simulink model "fullCarModel"  (R2024b)
settings: Solver=ode45  StartTime=0.0  StopTime=10.0  RelTol=1e-3  EnableMultiTasking=on
undefined symbols (not defined in the file or in its folder): sigbuilder_block
(part 2 of 2)

== system fullCarModel/vehicleBodyWith4Wheels/FullVehicle/wheelFR/FxfN/alfaFrontNew ==
  delta : Inport
  yVelo : Inport  Port=2
  Lf : Inport  Port=3
  yawRate : Inport  Port=4
  xVelo : Inport  Port=5
  Add : Sum  Inputs=+-
  Add1 : Sum
  Divide : Product  Inputs=*/
  Product : Product  RndMeth=Zero
  alfaFront : Outport
  wires:
  Lf/1 -> Product/1
  yawRate/1 -> Product/2
  Product/1 -> Add1/2
  yVelo/1 -> Add1/1
  Add1/1 -> Divide/1
  Divide/1 -> Add/2
  delta/1 -> Add/1
  Add/1 -> alfaFront/1
  xVelo/1 -> Divide/2

== system fullCarModel/vehicleBodyWith4Wheels/FullVehicle/wheelFR/FxfN/fLemda ==
  lamda : Inport
  Add : Sum  Inputs=+-
  Constant : Constant  Value=2
  Constant1 : Constant
  If : If  IfExpression=u1< 1  ZeroCross=off
  If Action Subsystem : Subsystem  TreatAsAtomicUnit=on
  If Action Subsystem1 : Subsystem  TreatAsAtomicUnit=on
  Merge : Merge
  Product : Product  RndMeth=Zero
  f_lamda : Outport
  wires:
  lamda/1 -> If/1, Add/2, Product/2
  If/1 -> If Action Subsystem1/Action
  If/2 -> If Action Subsystem/Action
  Constant/1 -> Add/1
  Add/1 -> Product/1
  Product/1 -> If Action Subsystem1/1(In1)
  Constant1/1 -> If Action Subsystem/1(In1)
  If Action Subsystem1/1(Out1) -> Merge/1
  If Action Subsystem/1(Out1) -> Merge/2
  Merge/1 -> f_lamda/1

== system fullCarModel/vehicleBodyWith4Wheels/FullVehicle/wheelFR/FxfN/lemda1 ==
  miu : Inport
  Fz : Inport  Port=2
  C_sigma : Inport  Port=3
  C_alfa : Inport  Port=4
  sigma : Inport  Port=5
  alfa : Inport  Port=6
  Add : Sum
  Add1 : Sum
  Constant : Constant  Value=2
  Constant1 : Constant
  Divide : Product  Inputs=*/
  Math Function : Math  Operator=square  SignedPower=on
  Math Function1 : Math  Operator=square  SignedPower=on
  Product{,1..4} (5 alike) : Product  RndMeth=Zero
  Sqrt : Sqrt
  Trigonometric Function : Trigonometry  Operator=tan
  lamda : Outport
  wires:
  C_alfa/1 -> Product1/1
  alfa/1 -> Trigonometric Function/1
  Trigonometric Function/1 -> Product1/2
  Product/1 -> Math Function/1
  Product1/1 -> Math Function1/1
  Math Function/1 -> Add/1
  Math Function1/1 -> Add/2
  Add/1 -> Sqrt/1
  Sqrt/1 -> Product2/1
  Constant/1 -> Product2/2
  C_sigma/1 -> Product/2
  sigma/1 -> Product/1, Add1/1
  miu/1 -> Product3/1
  Fz/1 -> Product3/2
  Constant1/1 -> Add1/2
  Product3/1 -> Product4/1
  Add1/1 -> Product4/2
  Product4/1 -> Divide/1
  Product2/1 -> Divide/2
  Divide/1 -> lamda/1

== system fullCarModel/vehicleBodyWith4Wheels/FullVehicle/wheelFR/FxfN/sigmaAccX2 ==
  reff : Inport
  w : Inport  Port=2
  Vx : Inport  Port=3
  Add : Sum  Inputs=+-
  Constant : Constant  Value=0
  Divide : Product  Inputs=*/
  If Action Subsystem2 : Subsystem  TreatAsAtomicUnit=on
  If Action Subsystem3 : Subsystem  TreatAsAtomicUnit=on
  If1 : If
  Merge1 : Merge
  Product : Product  RndMeth=Zero
  sigmaAccX : Outport
  wires:
  reff/1 -> Product/1
  Product/1 -> Add/1, Divide/2
  Add/1 -> Divide/1
  w/1 -> Product/2
  Vx/1 -> Add/2
  Divide/1 -> If Action Subsystem2/1(In1), If1/1
  If1/1 -> If Action Subsystem2/Action
  If1/2 -> If Action Subsystem3/Action
  If Action Subsystem2/1(Out1) -> Merge1/1
  If Action Subsystem3/1(Out1) -> Merge1/2
  Constant/1 -> If Action Subsystem3/1(In1)
  Merge1/1 -> sigmaAccX/1

== system fullCarModel/vehicleBodyWith4Wheels/FullVehicle/wheelFR/FyfN/alfaFrontNew ==
  delta : Inport
  yVelo : Inport  Port=2
  Lf : Inport  Port=3
  yawRate : Inport  Port=4
  xVelo : Inport  Port=5
  Add : Sum  Inputs=+-
  Add1 : Sum
  Divide : Product  Inputs=*/
  Product : Product  RndMeth=Zero
  alfaFront : Outport
  wires:
  Lf/1 -> Product/1
  yawRate/1 -> Product/2
  Product/1 -> Add1/2
  yVelo/1 -> Add1/1
  Add1/1 -> Divide/1
  Divide/1 -> Add/2
  delta/1 -> Add/1
  Add/1 -> alfaFront/1
  xVelo/1 -> Divide/2

== system fullCarModel/vehicleBodyWith4Wheels/FullVehicle/wheelFR/FyfN/f_lamda ==
  lamda : Inport
  Add : Sum  Inputs=+-
  Constant : Constant  Value=2
  Constant1 : Constant
  If : If  IfExpression=u1< 1  ZeroCross=off
  If Action Subsystem : Subsystem  TreatAsAtomicUnit=on
  If Action Subsystem1 : Subsystem  TreatAsAtomicUnit=on
  Merge : Merge
  Product : Product  RndMeth=Zero
  f_lamda : Outport
  wires:
  lamda/1 -> If/1, Add/2, Product/2
  If/1 -> If Action Subsystem1/Action
  If/2 -> If Action Subsystem/Action
  Constant/1 -> Add/1
  Add/1 -> Product/1
  Product/1 -> If Action Subsystem1/1(In1)
  Constant1/1 -> If Action Subsystem/1(In1)
  If Action Subsystem1/1(Out1) -> Merge/1
  If Action Subsystem/1(Out1) -> Merge/2
  Merge/1 -> f_lamda/1

== system fullCarModel/vehicleBodyWith4Wheels/FullVehicle/wheelFR/FyfN/lemda1 ==
  miu : Inport
  Fz : Inport  Port=2
  C_sigma : Inport  Port=3
  C_alfa : Inport  Port=4
  sigma : Inport  Port=5
  alfa : Inport  Port=6
  Add : Sum
  Add1 : Sum
  Constant : Constant  Value=2
  Constant1 : Constant
  Divide : Product  Inputs=*/
  Math Function : Math  Operator=square  SignedPower=on
  Math Function1 : Math  Operator=square  SignedPower=on
  Product{,1..4} (5 alike) : Product  RndMeth=Zero
  Sqrt : Sqrt
  Trigonometric Function : Trigonometry  Operator=tan
  lamda : Outport
  wires:
  C_alfa/1 -> Product1/1
  alfa/1 -> Trigonometric Function/1
  Trigonometric Function/1 -> Product1/2
  Product/1 -> Math Function/1
  Product1/1 -> Math Function1/1
  Math Function/1 -> Add/1
  Math Function1/1 -> Add/2
  Add/1 -> Sqrt/1
  Sqrt/1 -> Product2/1
  Constant/1 -> Product2/2
  C_sigma/1 -> Product/2
  sigma/1 -> Product/1, Add1/1
  miu/1 -> Product3/1
  Fz/1 -> Product3/2
  Constant1/1 -> Add1/2
  Product3/1 -> Product4/1
  Add1/1 -> Product4/2
  Product4/1 -> Divide/1
  Product2/1 -> Divide/2
  Divide/1 -> lamda/1

== system fullCarModel/vehicleBodyWith4Wheels/FullVehicle/wheelFR/FyfN/sigmaAccX2 ==
  reff : Inport
  w : Inport  Port=2
  Vx : Inport  Port=3
  Add : Sum  Inputs=+-
  Constant : Constant  Value=0
  Divide : Product  Inputs=*/
  If Action Subsystem2 : Subsystem  TreatAsAtomicUnit=on
  If Action Subsystem3 : Subsystem  TreatAsAtomicUnit=on
  If1 : If
  Merge1 : Merge
  Product : Product  RndMeth=Zero
  sigmaAccX : Outport
  wires:
  reff/1 -> Product/1
  Product/1 -> Add/1, Divide/2
  Add/1 -> Divide/1
  w/1 -> Product/2
  Vx/1 -> Add/2
  Divide/1 -> If Action Subsystem2/1(In1), If1/1
  If1/1 -> If Action Subsystem2/Action
  If1/2 -> If Action Subsystem3/Action
  If Action Subsystem2/1(Out1) -> Merge1/1
  If Action Subsystem3/1(Out1) -> Merge1/2
  Constant/1 -> If Action Subsystem3/1(In1)
  Merge1/1 -> sigmaAccX/1

== system fullCarModel/vehicleBodyWith4Wheels/FullVehicle/wheel_RL/FxrN/alfaRearNew ==
  yVelo : Inport
  Lr : Inport  Port=2
  yawRate : Inport  Port=3
  xVelo : Inport  Port=4
  Add1 : Sum  Inputs=+-
  Divide : Product  Inputs=*/
  Gain : Gain  Gain=-1
  Product : Product  RndMeth=Zero
  alfaRear : Outport
  wires:
  Lr/1 -> Product/1
  yawRate/1 -> Product/2
  Product/1 -> Add1/2
  yVelo/1 -> Add1/1
  Add1/1 -> Divide/1
  Divide/1 -> Gain/1
  Gain/1 -> alfaRear/1
  xVelo/1 -> Divide/2

== system fullCarModel/vehicleBodyWith4Wheels/FullVehicle/wheel_RL/FxrN/f_lamda ==
  lamda : Inport
  Add : Sum  Inputs=+-
  Constant : Constant  Value=2
  Constant1 : Constant
  If : If  IfExpression=u1< 1  ZeroCross=off
  If Action Subsystem : Subsystem  TreatAsAtomicUnit=on
  If Action Subsystem1 : Subsystem  TreatAsAtomicUnit=on
  Merge : Merge
  Product : Product  RndMeth=Zero
  f_lamda : Outport
  wires:
  lamda/1 -> If/1, Add/2, Product/2
  If/1 -> If Action Subsystem1/Action
  If/2 -> If Action Subsystem/Action
  Constant/1 -> Add/1
  Add/1 -> Product/1
  Product/1 -> If Action Subsystem1/1(In1)
  Constant1/1 -> If Action Subsystem/1(In1)
  If Action Subsystem1/1(Out1) -> Merge/1
  If Action Subsystem/1(Out1) -> Merge/2
  Merge/1 -> f_lamda/1

== system fullCarModel/vehicleBodyWith4Wheels/FullVehicle/wheel_RL/FxrN/lemda1 ==
  miu : Inport
  Fz : Inport  Port=2
  C_sigma : Inport  Port=3
  C_alfa : Inport  Port=4
  sigma : Inport  Port=5
  alfa : Inport  Port=6
  Add : Sum
  Add1 : Sum
  Constant : Constant  Value=2
  Constant1 : Constant
  Divide : Product  Inputs=*/
  Math Function : Math  Operator=square  SignedPower=on
  Math Function1 : Math  Operator=square  SignedPower=on
  Product{,1..4} (5 alike) : Product  RndMeth=Zero
  Sqrt : Sqrt
  Trigonometric Function : Trigonometry  Operator=tan
  lamda : Outport
  wires:
  C_alfa/1 -> Product1/1
  alfa/1 -> Trigonometric Function/1
  Trigonometric Function/1 -> Product1/2
  Product/1 -> Math Function/1
  Product1/1 -> Math Function1/1
  Math Function/1 -> Add/1
  Math Function1/1 -> Add/2
  Add/1 -> Sqrt/1
  Sqrt/1 -> Product2/1
  Constant/1 -> Product2/2
  C_sigma/1 -> Product/2
  sigma/1 -> Product/1, Add1/1
  miu/1 -> Product3/1
  Fz/1 -> Product3/2
  Constant1/1 -> Add1/2
  Product3/1 -> Product4/1
  Add1/1 -> Product4/2
  Product4/1 -> Divide/1
  Product2/1 -> Divide/2
  Divide/1 -> lamda/1

== system fullCarModel/vehicleBodyWith4Wheels/FullVehicle/wheel_RL/FxrN/sigmaAccX2 ==
  reff : Inport
  w : Inport  Port=2
  Vx : Inport  Port=3
  Add : Sum  Inputs=+-
  Constant : Constant  Value=0
  Divide : Product  Inputs=*/
  If Action Subsystem2 : Subsystem  TreatAsAtomicUnit=on
  If Action Subsystem3 : Subsystem  TreatAsAtomicUnit=on
  If1 : If
  Merge1 : Merge
  Product : Product  RndMeth=Zero
  sigmaAccX : Outport
  wires:
  reff/1 -> Product/1
  Product/1 -> Add/1, Divide/2
  Add/1 -> Divide/1
  w/1 -> Product/2
  Vx/1 -> Add/2
  Divide/1 -> If Action Subsystem2/1(In1), If1/1
  If1/1 -> If Action Subsystem2/Action
  If1/2 -> If Action Subsystem3/Action
  If Action Subsystem2/1(Out1) -> Merge1/1
  If Action Subsystem3/1(Out1) -> Merge1/2
  Constant/1 -> If Action Subsystem3/1(In1)
  Merge1/1 -> sigmaAccX/1

== system fullCarModel/vehicleBodyWith4Wheels/FullVehicle/wheel_RL/FyrN/alfaRearNew ==
  yVelo : Inport
  Lr : Inport  Port=2
  yawRate : Inport  Port=3
  xVelo : Inport  Port=4
  Add1 : Sum  Inputs=+-
  Divide : Product  Inputs=*/
  Gain : Gain  Gain=-1
  Product : Product  RndMeth=Zero
  alfaRear : Outport
  wires:
  Lr/1 -> Product/1
  yawRate/1 -> Product/2
  Product/1 -> Add1/2
  yVelo/1 -> Add1/1
  Add1/1 -> Divide/1
  Divide/1 -> Gain/1
  Gain/1 -> alfaRear/1
  xVelo/1 -> Divide/2

== system fullCarModel/vehicleBodyWith4Wheels/FullVehicle/wheel_RL/FyrN/f_lamda ==
  lamda : Inport
  Add : Sum  Inputs=+-
  Constant : Constant  Value=2
  Constant1 : Constant
  If : If  IfExpression=u1< 1  ZeroCross=off
  If Action Subsystem : Subsystem  TreatAsAtomicUnit=on
  If Action Subsystem1 : Subsystem  TreatAsAtomicUnit=on
  Merge : Merge
  Product : Product  RndMeth=Zero
  f_lamda : Outport
  wires:
  lamda/1 -> If/1, Add/2, Product/2
  If/1 -> If Action Subsystem1/Action
  If/2 -> If Action Subsystem/Action
  Constant/1 -> Add/1
  Add/1 -> Product/1
  Product/1 -> If Action Subsystem1/1(In1)
  Constant1/1 -> If Action Subsystem/1(In1)
  If Action Subsystem1/1(Out1) -> Merge/1
  If Action Subsystem/1(Out1) -> Merge/2
  Merge/1 -> f_lamda/1

== system fullCarModel/vehicleBodyWith4Wheels/FullVehicle/wheel_RL/FyrN/lemda1 ==
  miu : Inport
  Fz : Inport  Port=2
  C_sigma : Inport  Port=3
  C_alfa : Inport  Port=4
  sigma : Inport  Port=5
  alfa : Inport  Port=6
  Add : Sum
  Add1 : Sum
  Constant : Constant  Value=2
  Constant1 : Constant
  Divide : Product  Inputs=*/
  Math Function : Math  Operator=square  SignedPower=on
  Math Function1 : Math  Operator=square  SignedPower=on
  Product{,1..4} (5 alike) : Product  RndMeth=Zero
  Sqrt : Sqrt
  Trigonometric Function : Trigonometry  Operator=tan
  lamda : Outport
  wires:
  C_alfa/1 -> Product1/1
  alfa/1 -> Trigonometric Function/1
  Trigonometric Function/1 -> Product1/2
  Product/1 -> Math Function/1
  Product1/1 -> Math Function1/1
  Math Function/1 -> Add/1
  Math Function1/1 -> Add/2
  Add/1 -> Sqrt/1
  Sqrt/1 -> Product2/1
  Constant/1 -> Product2/2
  C_sigma/1 -> Product/2
  sigma/1 -> Product/1, Add1/1
  miu/1 -> Product3/1
  Fz/1 -> Product3/2
  Constant1/1 -> Add1/2
  Product3/1 -> Product4/1
  Add1/1 -> Product4/2
  Product4/1 -> Divide/1
  Product2/1 -> Divide/2
  Divide/1 -> lamda/1

== system fullCarModel/vehicleBodyWith4Wheels/FullVehicle/wheel_RL/FyrN/sigmaAccX2 ==
  reff : Inport
  w : Inport  Port=2
  Vx : Inport  Port=3
  Add : Sum  Inputs=+-
  Constant : Constant  Value=0
  Divide : Product  Inputs=*/
  If Action Subsystem2 : Subsystem  TreatAsAtomicUnit=on
  If Action Subsystem3 : Subsystem  TreatAsAtomicUnit=on
  If1 : If
  Merge1 : Merge
  Product : Product  RndMeth=Zero
  sigmaAccX : Outport
  wires:
  reff/1 -> Product/1
  Product/1 -> Add/1, Divide/2
  Add/1 -> Divide/1
  w/1 -> Product/2
  Vx/1 -> Add/2
  Divide/1 -> If Action Subsystem2/1(In1), If1/1
  If1/1 -> If Action Subsystem2/Action
  If1/2 -> If Action Subsystem3/Action
  If Action Subsystem2/1(Out1) -> Merge1/1
  If Action Subsystem3/1(Out1) -> Merge1/2
  Constant/1 -> If Action Subsystem3/1(In1)
  Merge1/1 -> sigmaAccX/1

== system fullCarModel/vehicleBodyWith4Wheels/FullVehicle/wheel_RR/FxrN/alfaRearNew ==
  yVelo : Inport
  Lr : Inport  Port=2
  yawRate : Inport  Port=3
  xVelo : Inport  Port=4
  Add1 : Sum  Inputs=+-
  Divide : Product  Inputs=*/
  Gain : Gain  Gain=-1
  Product : Product  RndMeth=Zero
  alfaRear : Outport
  wires:
  Lr/1 -> Product/1
  yawRate/1 -> Product/2
  Product/1 -> Add1/2
  yVelo/1 -> Add1/1
  Add1/1 -> Divide/1
  Divide/1 -> Gain/1
  Gain/1 -> alfaRear/1
  xVelo/1 -> Divide/2

== system fullCarModel/vehicleBodyWith4Wheels/FullVehicle/wheel_RR/FxrN/f_lamda ==
  lamda : Inport
  Add : Sum  Inputs=+-
  Constant : Constant  Value=2
  Constant1 : Constant
  If : If  IfExpression=u1< 1  ZeroCross=off
  If Action Subsystem : Subsystem  TreatAsAtomicUnit=on
  If Action Subsystem1 : Subsystem  TreatAsAtomicUnit=on
  Merge : Merge
  Product : Product  RndMeth=Zero
  f_lamda : Outport
  wires:
  lamda/1 -> If/1, Add/2, Product/2
  If/1 -> If Action Subsystem1/Action
  If/2 -> If Action Subsystem/Action
  Constant/1 -> Add/1
  Add/1 -> Product/1
  Product/1 -> If Action Subsystem1/1(In1)
  Constant1/1 -> If Action Subsystem/1(In1)
  If Action Subsystem1/1(Out1) -> Merge/1
  If Action Subsystem/1(Out1) -> Merge/2
  Merge/1 -> f_lamda/1

== system fullCarModel/vehicleBodyWith4Wheels/FullVehicle/wheel_RR/FxrN/lemda1 ==
  miu : Inport
  Fz : Inport  Port=2
  C_sigma : Inport  Port=3
  C_alfa : Inport  Port=4
  sigma : Inport  Port=5
  alfa : Inport  Port=6
  Add : Sum
  Add1 : Sum
  Constant : Constant  Value=2
  Constant1 : Constant
  Divide : Product  Inputs=*/
  Math Function : Math  Operator=square  SignedPower=on
  Math Function1 : Math  Operator=square  SignedPower=on
  Product{,1..4} (5 alike) : Product  RndMeth=Zero
  Scope : Scope
  Scope2 : Scope
  Sqrt : Sqrt
  Trigonometric Function : Trigonometry  Operator=tan
  lamda : Outport
  wires:
  C_alfa/1 -> Product1/1
  alfa/1 -> Trigonometric Function/1
  Trigonometric Function/1 -> Product1/2
  Product/1 -> Math Function/1
  Product1/1 -> Math Function1/1
  Math Function/1 -> Add/1
  Math Function1/1 -> Add/2
  Add/1 -> Scope2/1, Sqrt/1
  Sqrt/1 -> Product2/1
  Constant/1 -> Product2/2
  C_sigma/1 -> Product/2
  sigma/1 -> Product/1, Add1/1
  miu/1 -> Product3/1
  Fz/1 -> Product3/2
  Constant1/1 -> Add1/2
  Product3/1 -> Product4/1
  Add1/1 -> Product4/2
  Product4/1 -> Divide/1
  Product2/1 -> Scope/1, Divide/2
  Divide/1 -> lamda/1

== system fullCarModel/vehicleBodyWith4Wheels/FullVehicle/wheel_RR/FxrN/sigmaAccX2 ==
  reff : Inport
  w : Inport  Port=2
  Vx : Inport  Port=3
  Add : Sum  Inputs=+-
  Constant : Constant  Value=0
  Divide : Product  Inputs=*/
  If Action Subsystem2 : Subsystem  TreatAsAtomicUnit=on
  If Action Subsystem3 : Subsystem  TreatAsAtomicUnit=on
  If1 : If
  Merge1 : Merge
  Product : Product  RndMeth=Zero
  sigmaAccX : Outport
  wires:
  reff/1 -> Product/1
  Product/1 -> Add/1, Divide/2
  Add/1 -> Divide/1
  w/1 -> Product/2
  Vx/1 -> Add/2
  Divide/1 -> If Action Subsystem2/1(In1), If1/1
  If1/1 -> If Action Subsystem2/Action
  If1/2 -> If Action Subsystem3/Action
  If Action Subsystem2/1(Out1) -> Merge1/1
  If Action Subsystem3/1(Out1) -> Merge1/2
  Constant/1 -> If Action Subsystem3/1(In1)
  Merge1/1 -> sigmaAccX/1

== system fullCarModel/vehicleBodyWith4Wheels/FullVehicle/wheel_RR/FyrN/alfaRearNew ==
  yVelo : Inport
  Lr : Inport  Port=2
  yawRate : Inport  Port=3
  xVelo : Inport  Port=4
  Add1 : Sum  Inputs=+-
  Divide : Product  Inputs=*/
  Gain : Gain  Gain=-1
  Product : Product  RndMeth=Zero
  alfaRear : Outport
  wires:
  Lr/1 -> Product/1
  yawRate/1 -> Product/2
  Product/1 -> Add1/2
  yVelo/1 -> Add1/1
  Add1/1 -> Divide/1
  Divide/1 -> Gain/1
  Gain/1 -> alfaRear/1
  xVelo/1 -> Divide/2

== system fullCarModel/vehicleBodyWith4Wheels/FullVehicle/wheel_RR/FyrN/f_lamda ==
  lamda : Inport
  Add : Sum  Inputs=+-
  Constant : Constant  Value=2
  Constant1 : Constant
  If : If  IfExpression=u1< 1  ZeroCross=off
  If Action Subsystem : Subsystem  TreatAsAtomicUnit=on
  If Action Subsystem1 : Subsystem  TreatAsAtomicUnit=on
  Merge : Merge
  Product : Product  RndMeth=Zero
  f_lamda : Outport
  wires:
  lamda/1 -> If/1, Add/2, Product/2
  If/1 -> If Action Subsystem1/Action
  If/2 -> If Action Subsystem/Action
  Constant/1 -> Add/1
  Add/1 -> Product/1
  Product/1 -> If Action Subsystem1/1(In1)
  Constant1/1 -> If Action Subsystem/1(In1)
  If Action Subsystem1/1(Out1) -> Merge/1
  If Action Subsystem/1(Out1) -> Merge/2
  Merge/1 -> f_lamda/1

== system fullCarModel/vehicleBodyWith4Wheels/FullVehicle/wheel_RR/FyrN/lemda1 ==
  miu : Inport
  Fz : Inport  Port=2
  C_sigma : Inport  Port=3
  C_alfa : Inport  Port=4
  sigma : Inport  Port=5
  alfa : Inport  Port=6
  Add : Sum
  Add1 : Sum
  Constant : Constant  Value=2
  Constant1 : Constant
  Divide : Product  Inputs=*/
  Math Function : Math  Operator=square  SignedPower=on
  Math Function1 : Math  Operator=square  SignedPower=on
  Product{,1..4} (5 alike) : Product  RndMeth=Zero
  Sqrt : Sqrt
  Trigonometric Function : Trigonometry  Operator=tan
  lamda : Outport
  wires:
  C_alfa/1 -> Product1/1
  alfa/1 -> Trigonometric Function/1
  Trigonometric Function/1 -> Product1/2
  Product/1 -> Math Function/1
  Product1/1 -> Math Function1/1
  Math Function/1 -> Add/1
  Math Function1/1 -> Add/2
  Add/1 -> Sqrt/1
  Sqrt/1 -> Product2/1
  Constant/1 -> Product2/2
  C_sigma/1 -> Product/2
  sigma/1 -> Product/1, Add1/1
  miu/1 -> Product3/1
  Fz/1 -> Product3/2
  Constant1/1 -> Add1/2
  Product3/1 -> Product4/1
  Add1/1 -> Product4/2
  Product4/1 -> Divide/1
  Product2/1 -> Divide/2
  Divide/1 -> lamda/1

== system fullCarModel/vehicleBodyWith4Wheels/FullVehicle/wheel_RR/FyrN/sigmaAccX2 ==
  reff : Inport
  w : Inport  Port=2
  Vx : Inport  Port=3
  Add : Sum  Inputs=+-
  Constant : Constant  Value=0
  Divide : Product  Inputs=*/
  If Action Subsystem2 : Subsystem  TreatAsAtomicUnit=on
  If Action Subsystem3 : Subsystem  TreatAsAtomicUnit=on
  If1 : If
  Merge1 : Merge
  Product : Product  RndMeth=Zero
  sigmaAccX : Outport
  wires:
  reff/1 -> Product/1
  Product/1 -> Add/1, Divide/2
  Add/1 -> Divide/1
  w/1 -> Product/2
  Vx/1 -> Add/2
  Divide/1 -> If Action Subsystem2/1(In1), If1/1
  If1/1 -> If Action Subsystem2/Action
  If1/2 -> If Action Subsystem3/Action
  If Action Subsystem2/1(Out1) -> Merge1/1
  If Action Subsystem3/1(Out1) -> Merge1/2
  Constant/1 -> If Action Subsystem3/1(In1)
  Merge1/1 -> sigmaAccX/1

== system fullCarModel/vehicleBodyWith4Wheels/FullVehicle/wheelFL/FxfN/fLemda/If Action Subsystem ==
  In1 : Inport
  Action Port : ActionPort  ActionPortLabel=else
  Out1 : Outport
  wires:
  In1/1 -> Out1/1

== system fullCarModel/vehicleBodyWith4Wheels/FullVehicle/wheelFL/FxfN/fLemda/If Action Subsystem1 ==
  In1 : Inport
  Action Port : ActionPort  ActionPortLabel=if(u1< 1)
  Out1 : Outport
  wires:
  In1/1 -> Out1/1

== system fullCarModel/vehicleBodyWith4Wheels/FullVehicle/wheelFL/FxfN/sigmaAccX2/If Action Subsystem2 ==
  In1 : Inport
  Action Port : ActionPort  ActionPortLabel=if(u1 > 0)
  Out1 : Outport
  wires:
  In1/1 -> Out1/1

== system fullCarModel/vehicleBodyWith4Wheels/FullVehicle/wheelFL/FxfN/sigmaAccX2/If Action Subsystem3 ==
  In1 : Inport
  Action Port : ActionPort  ActionPortLabel=else
  Out1 : Outport
  wires:
  In1/1 -> Out1/1

== system fullCarModel/vehicleBodyWith4Wheels/FullVehicle/wheelFL/FyfN/f_lamda/If Action Subsystem ==
  In1 : Inport
  Action Port : ActionPort  ActionPortLabel=else
  Out1 : Outport
  wires:
  In1/1 -> Out1/1

== system fullCarModel/vehicleBodyWith4Wheels/FullVehicle/wheelFL/FyfN/f_lamda/If Action Subsystem1 ==
  In1 : Inport
  Action Port : ActionPort  ActionPortLabel=if(u1< 1)
  Out1 : Outport
  wires:
  In1/1 -> Out1/1

== system fullCarModel/vehicleBodyWith4Wheels/FullVehicle/wheelFL/FyfN/sigmaAccX1/If Action Subsystem2 ==
  In1 : Inport
  Action Port : ActionPort  ActionPortLabel=if(u1 > 0)
  Out1 : Outport
  wires:
  In1/1 -> Out1/1

== system fullCarModel/vehicleBodyWith4Wheels/FullVehicle/wheelFL/FyfN/sigmaAccX1/If Action Subsystem3 ==
  In1 : Inport
  Action Port : ActionPort  ActionPortLabel=else
  Out1 : Outport
  wires:
  In1/1 -> Out1/1

== system fullCarModel/vehicleBodyWith4Wheels/FullVehicle/wheelFR/FxfN/fLemda/If Action Subsystem ==
  In1 : Inport
  Action Port : ActionPort  ActionPortLabel=else
  Out1 : Outport
  wires:
  In1/1 -> Out1/1

== system fullCarModel/vehicleBodyWith4Wheels/FullVehicle/wheelFR/FxfN/fLemda/If Action Subsystem1 ==
  In1 : Inport
  Action Port : ActionPort  ActionPortLabel=if(u1< 1)
  Out1 : Outport
  wires:
  In1/1 -> Out1/1

== system fullCarModel/vehicleBodyWith4Wheels/FullVehicle/wheelFR/FxfN/sigmaAccX2/If Action Subsystem2 ==
  In1 : Inport
  Action Port : ActionPort  ActionPortLabel=if(u1 > 0)
  Out1 : Outport
  wires:
  In1/1 -> Out1/1

== system fullCarModel/vehicleBodyWith4Wheels/FullVehicle/wheelFR/FxfN/sigmaAccX2/If Action Subsystem3 ==
  In1 : Inport
  Action Port : ActionPort  ActionPortLabel=else
  Out1 : Outport
  wires:
  In1/1 -> Out1/1

== system fullCarModel/vehicleBodyWith4Wheels/FullVehicle/wheelFR/FyfN/f_lamda/If Action Subsystem ==
  In1 : Inport
  Action Port : ActionPort  ActionPortLabel=else
  Out1 : Outport
  wires:
  In1/1 -> Out1/1

== system fullCarModel/vehicleBodyWith4Wheels/FullVehicle/wheelFR/FyfN/f_lamda/If Action Subsystem1 ==
  In1 : Inport
  Action Port : ActionPort  ActionPortLabel=if(u1< 1)
  Out1 : Outport
  wires:
  In1/1 -> Out1/1

== system fullCarModel/vehicleBodyWith4Wheels/FullVehicle/wheelFR/FyfN/sigmaAccX2/If Action Subsystem2 ==
  In1 : Inport
  Action Port : ActionPort  ActionPortLabel=if(u1 > 0)
  Out1 : Outport
  wires:
  In1/1 -> Out1/1

== system fullCarModel/vehicleBodyWith4Wheels/FullVehicle/wheelFR/FyfN/sigmaAccX2/If Action Subsystem3 ==
  In1 : Inport
  Action Port : ActionPort  ActionPortLabel=else
  Out1 : Outport
  wires:
  In1/1 -> Out1/1

== system fullCarModel/vehicleBodyWith4Wheels/FullVehicle/wheel_RL/FxrN/f_lamda/If Action Subsystem ==
  In1 : Inport
  Action Port : ActionPort  ActionPortLabel=else
  Out1 : Outport
  wires:
  In1/1 -> Out1/1

== system fullCarModel/vehicleBodyWith4Wheels/FullVehicle/wheel_RL/FxrN/f_lamda/If Action Subsystem1 ==
  In1 : Inport
  Action Port : ActionPort  ActionPortLabel=if(u1< 1)
  Out1 : Outport
  wires:
  In1/1 -> Out1/1

== system fullCarModel/vehicleBodyWith4Wheels/FullVehicle/wheel_RL/FxrN/sigmaAccX2/If Action Subsystem2 ==
  In1 : Inport
  Action Port : ActionPort  ActionPortLabel=if(u1 > 0)
  Out1 : Outport
  wires:
  In1/1 -> Out1/1

== system fullCarModel/vehicleBodyWith4Wheels/FullVehicle/wheel_RL/FxrN/sigmaAccX2/If Action Subsystem3 ==
  In1 : Inport
  Action Port : ActionPort  ActionPortLabel=else
  Out1 : Outport
  wires:
  In1/1 -> Out1/1

== system fullCarModel/vehicleBodyWith4Wheels/FullVehicle/wheel_RL/FyrN/f_lamda/If Action Subsystem ==
  In1 : Inport
  Action Port : ActionPort  ActionPortLabel=else
  Out1 : Outport
  wires:
  In1/1 -> Out1/1

== system fullCarModel/vehicleBodyWith4Wheels/FullVehicle/wheel_RL/FyrN/f_lamda/If Action Subsystem1 ==
  In1 : Inport
  Action Port : ActionPort  ActionPortLabel=if(u1< 1)
  Out1 : Outport
  wires:
  In1/1 -> Out1/1

== system fullCarModel/vehicleBodyWith4Wheels/FullVehicle/wheel_RL/FyrN/sigmaAccX2/If Action Subsystem2 ==
  In1 : Inport
  Action Port : ActionPort  ActionPortLabel=if(u1 > 0)
  Out1 : Outport
  wires:
  In1/1 -> Out1/1

== system fullCarModel/vehicleBodyWith4Wheels/FullVehicle/wheel_RL/FyrN/sigmaAccX2/If Action Subsystem3 ==
  In1 : Inport
  Action Port : ActionPort  ActionPortLabel=else
  Out1 : Outport
  wires:
  In1/1 -> Out1/1

== system fullCarModel/vehicleBodyWith4Wheels/FullVehicle/wheel_RR/FxrN/f_lamda/If Action Subsystem ==
  In1 : Inport
  Action Port : ActionPort  ActionPortLabel=else
  Out1 : Outport
  wires:
  In1/1 -> Out1/1

== system fullCarModel/vehicleBodyWith4Wheels/FullVehicle/wheel_RR/FxrN/f_lamda/If Action Subsystem1 ==
  In1 : Inport
  Action Port : ActionPort  ActionPortLabel=if(u1< 1)
  Out1 : Outport
  wires:
  In1/1 -> Out1/1

== system fullCarModel/vehicleBodyWith4Wheels/FullVehicle/wheel_RR/FxrN/sigmaAccX2/If Action Subsystem2 ==
  In1 : Inport
  Action Port : ActionPort  ActionPortLabel=if(u1 > 0)
  Out1 : Outport
  wires:
  In1/1 -> Out1/1

== system fullCarModel/vehicleBodyWith4Wheels/FullVehicle/wheel_RR/FxrN/sigmaAccX2/If Action Subsystem3 ==
  In1 : Inport
  Action Port : ActionPort  ActionPortLabel=else
  Out1 : Outport
  wires:
  In1/1 -> Out1/1

== system fullCarModel/vehicleBodyWith4Wheels/FullVehicle/wheel_RR/FyrN/f_lamda/If Action Subsystem ==
  In1 : Inport
  Action Port : ActionPort  ActionPortLabel=else
  Out1 : Outport
  wires:
  In1/1 -> Out1/1

== system fullCarModel/vehicleBodyWith4Wheels/FullVehicle/wheel_RR/FyrN/f_lamda/If Action Subsystem1 ==
  In1 : Inport
  Action Port : ActionPort  ActionPortLabel=if(u1< 1)
  Out1 : Outport
  wires:
  In1/1 -> Out1/1

== system fullCarModel/vehicleBodyWith4Wheels/FullVehicle/wheel_RR/FyrN/sigmaAccX2/If Action Subsystem2 ==
  In1 : Inport
  Action Port : ActionPort  ActionPortLabel=if(u1 > 0)
  Out1 : Outport
  wires:
  In1/1 -> Out1/1

== system fullCarModel/vehicleBodyWith4Wheels/FullVehicle/wheel_RR/FyrN/sigmaAccX2/If Action Subsystem3 ==
  In1 : Inport
  Action Port : ActionPort  ActionPortLabel=else
  Out1 : Outport
  wires:
  In1/1 -> Out1/1
